simulink model "math_lib"  (R2023a)
settings: configuration reference "config" (kept outside this file)
settings Model: DataDictionary=model_config.sldd  Creator=huangcheng  LastModifiedBy=Administrator
settings ConfigSetRef: SourceName=config

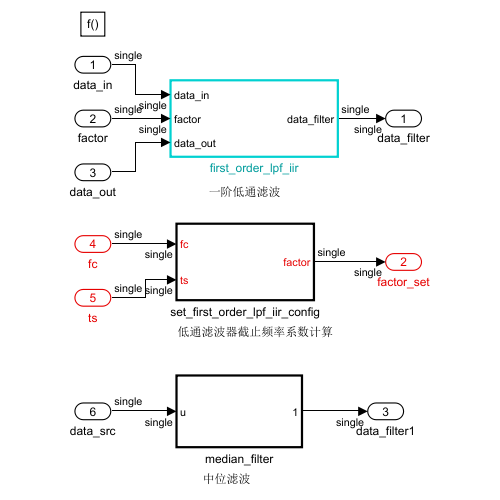
[thumbnail: Simulink's stored preview of the top-level diagram]
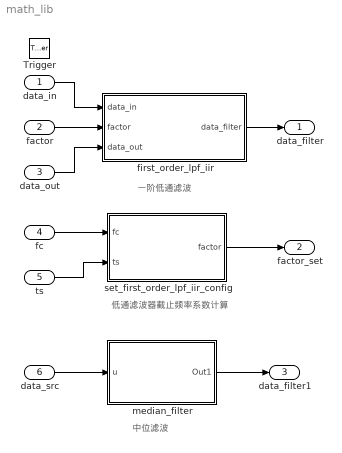
== system math_lib ==
  note: 低通滤波器截止频率系数计算
  note: 一阶低通滤波
  note: 中位滤波
  data_in : Inport  OutDataTypeStr=single
  factor : Inport  Port=2  OutMin=0  OutMax=1  OutDataTypeStr=single
  data_out : Inport  Port=3
  fc : Inport  Port=4  OutDataTypeStr=single
  ts : Inport  Port=5  OutDataTypeStr=single
  data_src : Inport  Port=6  OutDataTypeStr=single  PortDimensions=3
  Trigger : TriggerPort  TriggerType=function-call  VariantControl=(inherit)  PortDimensions=1
  first_order_lpf_iir : Subsystem  TreatAsAtomicUnit=on
  median_filter : Subsystem  TreatAsAtomicUnit=on
  set_first_order_lpf_iir_config : Subsystem  TreatAsAtomicUnit=on
  data_filter : Outport  OutDataTypeStr=single
  factor_set : Outport  Port=2  OutDataTypeStr=single
  data_filter1 : Outport  Port=3  OutDataTypeStr=single
  wires:
  data_in/1 -> first_order_lpf_iir/1(data_in)
  set_first_order_lpf_iir_config/1(factor) -> factor_set/1
  fc/1 -> set_first_order_lpf_iir_config/1(fc)
  factor/1 -> first_order_lpf_iir/2(factor)
  first_order_lpf_iir/1(data_filter) -> data_filter/1
  ts/1 -> set_first_order_lpf_iir_config/2(ts)
  data_out/1 -> first_order_lpf_iir/3(data_out)
  data_src/1 -> median_filter/1(u)
  median_filter/1(Out1) -> data_filter1/1

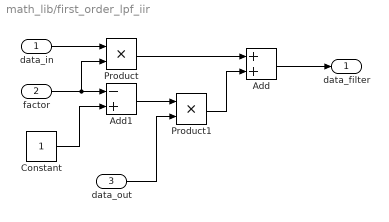
== system math_lib/first_order_lpf_iir ==
  data_in : Inport  OutDataTypeStr=single
  factor : Inport  Port=2  OutMin=0  OutMax=1  OutDataTypeStr=single
  data_out : Inport  Port=3
  Add : Sum
  Add1 : Sum  Inputs=-+
  Constant : Constant  OutDataTypeStr=single
  Product : Product
  Product1 : Product
  data_filter : Outport  OutDataTypeStr=single
  wires:
  Add/1 -> data_filter/1
  factor/1 -> Add1/1, Product/2
  Constant/1 -> Add1/2
  Product/1 -> Add/1
  data_in/1 -> Product/1
  Add1/1 -> Product1/1
  data_out/1 -> Product1/2
  Product1/1 -> Add/2

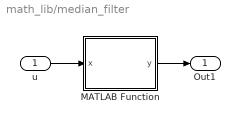
== system math_lib/median_filter ==
  u : Inport  OutDataTypeStr=single  PortDimensions=3
  MATLAB Function : MATLAB Function  TreatAsAtomicUnit=on
  Out1 : Outport
  wires:
  u/1 -> MATLAB Function/1(x)
  MATLAB Function/1(y) -> Out1/1

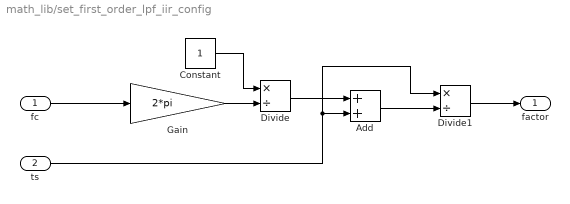
== system math_lib/set_first_order_lpf_iir_config ==
  fc : Inport  OutDataTypeStr=single
  ts : Inport  Port=2  OutDataTypeStr=single
  Add : Sum
  Constant : Constant  OutDataTypeStr=single
  Divide : Product  Inputs=*/
  Divide1 : Product  Inputs=*/
  Gain : Gain  Gain=2*pi
  factor : Outport  OutDataTypeStr=single
  wires:
  Divide/1 -> Add/1
  Gain/1 -> Divide/2
  ts/1 -> Add/2, Divide1/1
  Add/1 -> Divide1/2
  Divide1/1 -> factor/1
  Constant/1 -> Divide/1
  fc/1 -> Gain/1

== matlab function math_lib/median_filter/MATLAB Function ==
  data: x input; y output
function y = fcn(x)

y = median(x);
